simulink model "VEC"  (R2016a)
settings: Solver=ode45  SolverMode=SingleTasking  StartTime=0.0  StopTime=2000  FixedStep=0.001  RelTol=1e-5  AbsTol=1e-6
PostLoadFcn:
  | sldemo_fuelsys_data(bdroot,'initialize_data','orig','float');
model workspace (MAT data in the model file):
  PressEst = [0.806253176324 0.553142316929 0.37151500209 0.277667903103 0.220198954207 0.181288665766 0.153200000489 0.115431020872 0.0913067476324 0.0746519188607 0.0625231108324 0.0533383634277 ... (306 elements, 18x17)]
  PressVect = [0.05 0.1 0.15 0.2 0.25 0.3 0.35 0.4 0.45 0.5 0.55 0.6 0.65 0.7 0.75 0.8 0.85 0.9 0.95]
  PumpCon = [-0.0556348 -0.0022828 0.0256932 0.0435188 0.0562692 0.0661194857143 0.0741572 0.08697 0.0972452 0.106070342857 0.1139892 0.121303866667 ... (342 elements, 18x19)]
  RampRateKiX = [100 200 300 400 500 600]
  RampRateKiY = [0 0.2 0.4 0.6 0.8 1]
  RampRateKiZ = [0.012  0.024  0.036  0.048  0.06  0.072; 0.024  0.048  0.072  0.096  0.12  0.144; 0.036  0.072  0.108  0.144  0.18  0.216; 0.048  0.096  0.144  0.192  0.24  0.288; 0.06  0.12  0.18  0.24  0.3  0.36; 0.072  0.144  0.216  0.288  0.36  0.432]
  SpeedEst = [471.837839721 550.80940091 777.559313277 1080.9243499 1418.36795322 1769.7468768 2125.37309264 2480.20345067 2831.37796793 3177.14006959 3516.32917143 4064.90417867 ... (323 elements, 17x19)]
  SpeedVect = [50 75 100 125 150 175 200 250 300 350 400 450 500 600 700 800 900 1000]
  ThrotEst = [0 0 0 0 0 0 0 0 0 0 0 0 ... (342 elements, 18x19)]
  ThrotVect = [0 3 6 9 12 15 18 21 24 27 30 35 46 57 68 79 90]
  hys = 25
  max_ego = 1.2
  max_press = 0.95
  max_speed = 6000
  max_throt = 90
  min_press = 0.05
  min_speed = 50
  min_throt = 3
  st_range = 0.0001
  zero_thresh = 250
undefined symbols (not defined in the file): DiscIntNeverNeededParam, sld_FuelModes, sldvsubsys
libraries: simulink x4, simulink_extras x1
CloseFcn:
  | clear EngSensors u8En* s16En* sldemo_fuelsys_output
Description:
  | This is a model of a fuel control system where Stateflow(R) is used to handle the fault management of the system.
  | The system contains four separate sensors: a throttle sensor, a speed sensor, an oxygen sensor, and a pressure sensor.
  | Each of these sensors is represented by a parallel state in Stateflow.  Each parallel state contains two substates, a
  | normal state and a failed state (the exception being the oxygen sensor, which also contains a warmup state).
  | 
  | If any of the sensor readings is outside an acceptable range, then a fault is registered in Stateflow, and the
  | substate of the corresponding subsystem transitions to the failed state.  If a subsystem recovers, it can
  | transition back to the normal state.  The number of failures in the system at any given time is represented
  | in the Fail parallel state.
  | 
  | The last parallel state in the Stateflow chart is called Fueling_Mode.  This state regulates the oxygen to
  | fuel mixture ratio.  If a failure is detected, then the oxygen to fuel ratio is increased.  If multiple failures
  | are detected, then the fuel system is disabled until there are no longer multiple failures in the system.
settings Model: ModifiedByFormat=The MathWorks Inc.  NumberOfSteps=2  ExtModeTrigMode=oneshot  ExtModeArmWhenConnect=off  ExtModeAutoUpdateStatusClock=off  Creator=The MathWorks, Inc.  LastModifiedBy=The MathWorks Inc.
settings DataIOCC: SaveFormat=StructureWithTime  SaveOutput=off  SaveTime=off  SignalLoggingName=sldemo_fuelsys_output
settings OptimizationCC: DefaultParameterBehavior=Inlined  UseDivisionForNetSlopeComputation=UseDivisionForReciprocalsOfIntegersOnly  InlineInvariantSignals=on  EnhancedBackFolding=on  StrengthReduction=on  BooleansAsBitfields=on  PassReuseOutputArgsAs=Individual arguments  ExpressionDepthLimit=2147483647  ZeroExternalMemoryAtStartup=off  ZeroInternalMemoryAtStartup=off  NoFixptDivByZeroProtection=on  EfficientFloat2IntCast=on  OptimizeModelRefInitCode=on  LifeSpan=1
settings DebuggingCC: SignalInfNanChecking=error  SaveWithParameterizedLinksMsg=none  UnderspecifiedInitializationDetection=Classic  CheckExecutionContextPreStartOutputMsg=on  CheckExecutionContextRuntimeOutputMsg=on  IntegerOverflowMsg=none  ParameterDowncastMsg=warning  ParameterOverflowMsg=none  ParameterPrecisionLossMsg=none  UnderSpecifiedDataTypeMsg=warning  FcnCallInpInsideContextMsg=UseLocalSettings  UniqueDataStoreMsg=error  BusObjectLabelMismatch=error  AllowSymbolicDim=off  StateNameClashWarn=warning  StrictBusMsg=ErrorOnBusTreatedAsVector  IntegerSaturationMsg=none
settings HardwareCC: ProdBitPerPointer=32  ProdLargestAtomicFloat=None  ProdWordSize=32  ProdHWDeviceType=Specified
settings ModelReferenceCC: PropagateSignalLabelsOutOfModel=off
settings SFSimCC: SimParseCustomCode=off
settings RTWCC: SystemTargetFile=ert.tlc  TemplateMakefile=ert_default_tmf  Description=Real-Time Workshop Embedded Coder  GenerateReport=on  RTWVerbose=off  IncludeHyperlinkInReport=on  LaunchReport=on  GenerateTraceInfo=on  GenerateTraceReport=on  GenerateTraceReportSl=on  GenerateTraceReportSf=on  GenerateTraceReportEml=on
settings CodeAppCC: ForceParamTrailComments=on  IgnoreCustomStorageClasses=off  IgnoreTestpoints=on  SimulinkDataObjDesc=on  SFDataObjDesc=on  CustomSymbolStrGlobalVar=rt$N$M  CustomSymbolStrType=$N$M  CustomSymbolStrFcn=$N$M$F  CustomSymbolStrMacro=$N$M  InsertBlockDesc=on  InternalIdentifier=Classic  ReqsInCode=on
settings ERTTargetCC: GenerateSampleERTMain=on  IncludeMdlTerminateFcn=off  SupportAbsoluteTime=off  SupportNonFinite=off  SupportComplex=off  InlinedParameterPlacement=NonHierarchical  ERTCustomFileTemplate=example_file_process.tlc  ConvertIfToSwitch=off  SuppressUnreachableDefaultCases=off
settings ConfigComp: CovPath=/fuel_rate_control/control_logic  CovSFcnEnable=off

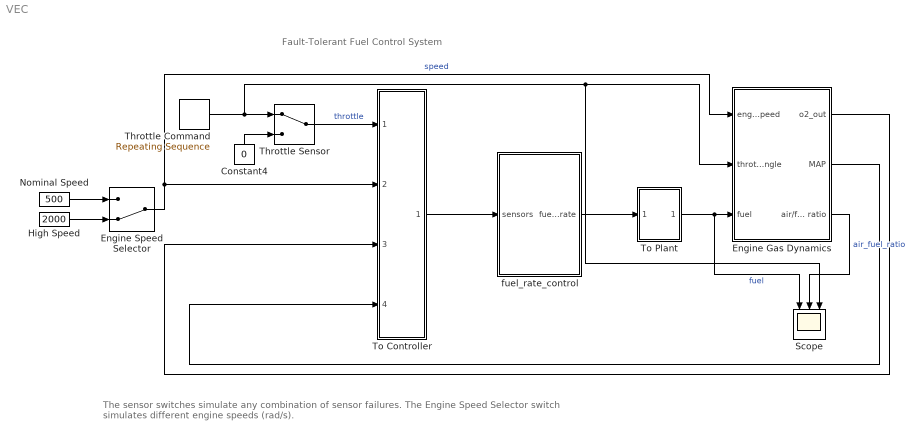
== system VEC ==
  note: Fault-Tolerant Fuel Control System
  note: The sensor switches simulate any combination of sensor failures.
      | The Engine Speed Selector switch simulates different engine speeds (rad/s).
  Constant4 : Constant  Value=0
  Engine Speed Selector : ManualSwitch  CurrentSetting=0
  Engine Gas Dynamics : Subsystem
  High Speed : Constant  Value=2000
  Nominal Speed : Constant  Value=500
  Scope : Scope  NumInputPorts=3
  Throttle Command : simulink/Sources/Repeating Sequence  rep_seq_t=[0 0.2 0.9 1]  rep_seq_y=[5 90 90 5]
  Throttle Sensor : ManualSwitch
  To Controller : Subsystem
      mask Display: fprintf('Convert')
  To Plant : Subsystem
      mask Display: fprintf('Convert')
  fuel_rate_control : Subsystem  Tag=FuelRateControl  TreatAsAtomicUnit=on
  wires:
  Engine Gas Dynamics/3(air/fuel ratio) -> Scope/2  "air_fuel_ratio"
  fuel_rate_control/1(fuel_rate) -> To Plant/1(In1)
  Engine Gas Dynamics/1(o2_out) -> To Controller/3(ego)
  Throttle Command/1 -> Scope/3, Engine Gas Dynamics/2(throttle angle), Throttle Sensor/1
  Constant4/1 -> Throttle Sensor/2
  Engine Gas Dynamics/2(MAP) -> To Controller/4(map)
  High Speed/1 -> Engine Speed Selector/2
  Nominal Speed/1 -> Engine Speed Selector/1
  Throttle Sensor/1 -> To Controller/1(throttle)  "throttle"
  Engine Speed Selector/1 -> To Controller/2(speed), Engine Gas Dynamics/1(engine speed)  "speed"
  To Plant/1(Out1) -> Scope/1, Engine Gas Dynamics/3(fuel)  "fuel"
  To Controller/1(sensors) -> fuel_rate_control/1(sensors)

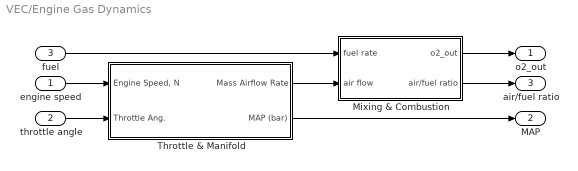
== system VEC/Engine Gas Dynamics ==
  engine speed : Inport  Unit=rad/s
  throttle angle : Inport  Port=2  Unit=deg
  fuel : Inport  Port=3  Unit=g/s
  Mixing & Combustion : Subsystem
  Throttle & Manifold : Subsystem
  o2_out : Outport  Unit=V
  MAP : Outport  Port=2  Unit=bar
  air/fuel ratio : Outport  Port=3  Unit=1
  wires:
  Throttle & Manifold/1(Mass Airflow Rate) -> Mixing & Combustion/2(air flow)
  fuel/1 -> Mixing & Combustion/1(fuel rate)
  engine speed/1 -> Throttle & Manifold/1("Engine Speed, N")
  throttle angle/1 -> Throttle & Manifold/2(Throttle Ang.)
  Mixing & Combustion/2(air/fuel ratio) -> air/fuel ratio/1
  Throttle & Manifold/2(MAP (bar)) -> MAP/1
  Mixing & Combustion/1(o2_out) -> o2_out/1

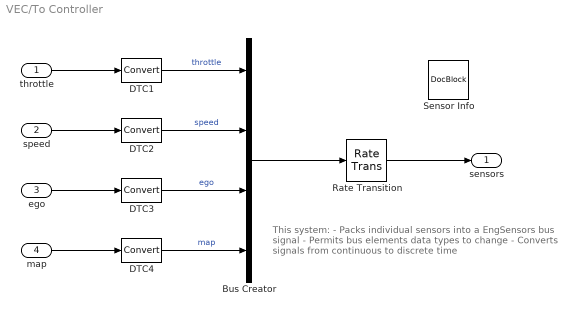
== system VEC/To Controller ==
  note: This system:
      | - Packs individual sensors into a EngSensors bus signal
      | - Permits bus elements data types to change
      | - Converts signals from continuous to discrete time
  throttle : Inport
  speed : Inport  Port=2
  ego : Inport  Port=3
  map : Inport  Port=4
  Bus Creator : BusCreator  Inputs=4  OutDataTypeStr=Bus: EngSensors  NonVirtualBus=on
  DTC{1..4} (4 alike) : DataTypeConversion  SampleTime=[0 1]
  Rate Transition : RateTransition  OutPortSampleTime=0.01
  Sensor Info : simulink/Model-Wide Utilities/DocBlock  DocumentType=Text
      content=|
      | Measurement Descriptions
      | ========================
      |
      | Throttle Angle (degrees):
      | min=3, max=90, precision=0.1
      |
      | Engine Speed (radians/sec.):
      | min=0, max=620, precision=.1
      |
      | Ego Sensor (volts):
      | min=0, max=12, precision=.05
      |
      | Manifold Pressure (bar):
      | min=0.001, max=1, precision=.001
  sensors : Outport
  wires:
  throttle/1 -> DTC1/1
  DTC1/1 -> Bus Creator/1  "throttle"
  speed/1 -> DTC2/1
  DTC2/1 -> Bus Creator/2  "speed"
  ego/1 -> DTC3/1
  DTC3/1 -> Bus Creator/3  "ego"
  map/1 -> DTC4/1
  DTC4/1 -> Bus Creator/4  "map"
  Bus Creator/1 -> Rate Transition/1
  Rate Transition/1 -> sensors/1

== system VEC/To Plant ==
  note: This system:
      | - Permits upstream signal data type to change
      | - Converts signals from discrete to continuous time
  In1 : Inport
  DTC5 : DataTypeConversion
  Rate Transition1 : RateTransition  Integrity=off  X0=1.6  OutPortSampleTime=0
  Out1 : Outport
  wires:
  DTC5/1 -> Rate Transition1/1
  In1/1 -> DTC5/1
  Rate Transition1/1 -> Out1/1

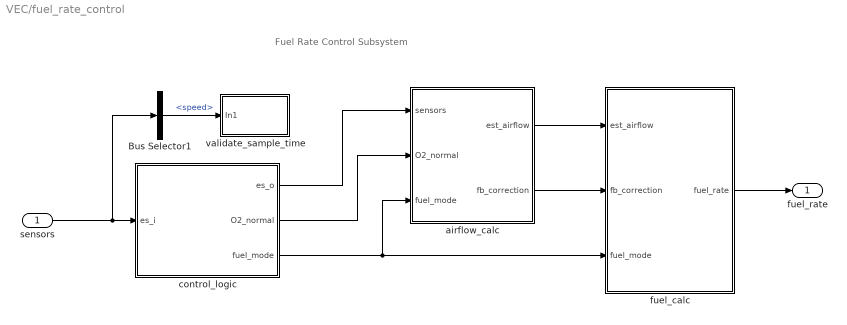
== system VEC/fuel_rate_control ==
  note: Fuel Rate Control Subsystem
  sensors : Inport  OutDataTypeStr=Bus: EngSensors
  Bus Selector1 : BusSelector  OutputSignals=speed
  airflow_calc : Subsystem
  control_logic : Stateflow chart  Description=Stateflow diagram to determine control system operating mode  TreatAsAtomicUnit=on
  fuel_calc : Subsystem
  validate_sample_time : Subsystem  Tag=VerificationSubsystem  DisableCoverage=on  LoadFcn=sldvsubsys('check')  TreatAsAtomicUnit=on  SimViewingDevice=on  mask(VerificationSubsystem){}
      mask init:
      | sldvsubsys('maskInit');
      settings: CopyFcn=sldvsubsys('copy');  OpenFcn=open_system(gcb,'force');
      settings: PreSaveFcn=|
      | set_param(gcb,'SimViewingDevice','on');
      | sldvsubsys('check');
      mask Help: helpview(fullfile(docroot,'toolbox','sldv','sldv.map'),'verificationsubsystem')
      mask Display: image(imread('sldvicon_versubsys.png','BackGroundColor',[1 1 1]),'center');
  fuel_rate : Outport  Unit=g/s
  wires:
  fuel_calc/1(fuel_rate) -> fuel_rate/1
  airflow_calc/1(est_airflow) -> fuel_calc/1(est_airflow)
  sensors/1 -> control_logic/1(es_i), Bus Selector1/1
  control_logic/3(fuel_mode) -> airflow_calc/3(fuel_mode), fuel_calc/3(fuel_mode)
  control_logic/1(es_o) -> airflow_calc/1(sensors)
  control_logic/2(" O2_normal") -> airflow_calc/2(O2_normal)
  airflow_calc/2(fb_correction) -> fuel_calc/2(fb_correction)
  Bus Selector1/1 -> validate_sample_time/1(In1)  "<speed>"

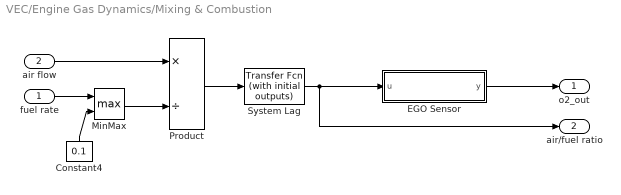
== system VEC/Engine Gas Dynamics/Mixing & Combustion ==
  fuel rate : Inport  Unit=g/s
  air flow : Inport  Port=2  Unit=g/s
  Constant4 : Constant  Value=0.1
  EGO Sensor : MATLAB Function  TreatAsAtomicUnit=on
  MinMax : MinMax  Function=max  Inputs=2  SaturateOnIntegerOverflow=on  InputSameDT=on
  Product : Product  Inputs=*/  SaturateOnIntegerOverflow=on  RndMeth=Zero  InputSameDT=on  OutDataTypeStr=Inherit: Same as first input
  System Lag : simulink_extras/Additional Linear/Transfer Fcn (with initial outputs)  N=3  D=[1 3]  Y0=1/14.6  U0=1/14.6
  o2_out : Outport  Unit=V
  air/fuel ratio : Outport  Port=2  Unit=1
  wires:
  Constant4/1 -> MinMax/2
  fuel rate/1 -> MinMax/1
  MinMax/1 -> Product/2
  Product/1 -> System Lag/1
  System Lag/1 -> air/fuel ratio/1, EGO Sensor/1(u)
  EGO Sensor/1(y) -> o2_out/1
  air flow/1 -> Product/1

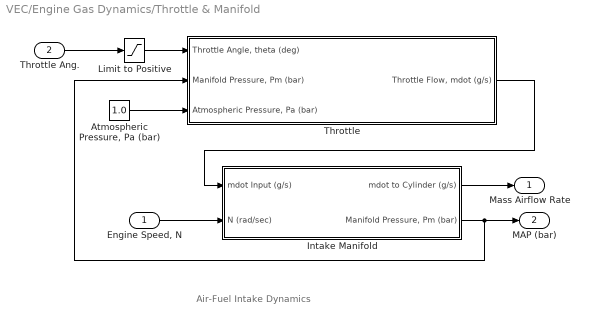
== system VEC/Engine Gas Dynamics/Throttle & Manifold ==
  note: Air-Fuel Intake Dynamics
  "Engine Speed, N" : Inport  Unit=rad/s
  Throttle Ang. : Inport  Port=2  Unit=deg
  "Atmospheric Pressure, Pa (bar)" : Constant  Value=1.0
  Intake Manifold : Subsystem
  Limit to Positive : Saturate  UpperLimit=inf  LowerLimit=0
  Throttle : Subsystem
  Mass Airflow Rate : Outport  Unit=g/s
  MAP (bar) : Outport  Port=2  Unit=bar
  wires:
  Limit to Positive/1 -> Throttle/1("Throttle Angle, theta (deg)")
  Throttle Ang./1 -> Limit to Positive/1
  Throttle/1("Throttle Flow, mdot (g/s)") -> Intake Manifold/1(mdot Input (g/s))
  "Engine Speed, N"/1 -> Intake Manifold/2(N (rad/sec))
  Intake Manifold/1(mdot to Cylinder (g/s)) -> Mass Airflow Rate/1
  "Atmospheric Pressure, Pa (bar)"/1 -> Throttle/3("Atmospheric Pressure, Pa (bar) ")
  Intake Manifold/2("Manifold Pressure, Pm (bar)") -> Throttle/2("Manifold Pressure, Pm (bar)"), MAP (bar)/1

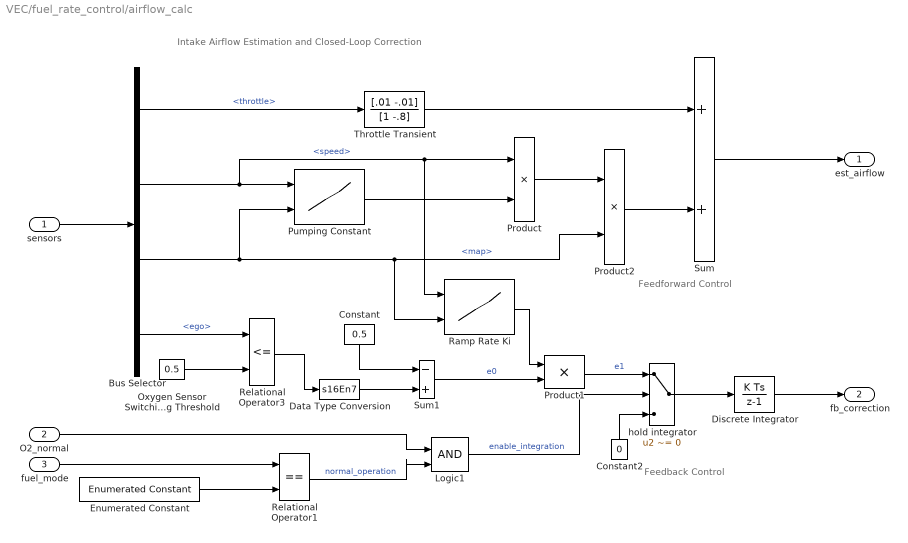
== system VEC/fuel_rate_control/airflow_calc ==
  note: Intake Airflow Estimation and Closed-Loop Correction
  note: Feedback Control
  note: Feedforward Control
  sensors : Inport
  O2_normal : Inport  Port=2
  fuel_mode : Inport  Port=3
  Bus Selector : BusSelector  OutputSignals=throttle,speed,map,ego
  Constant : Constant  Value=0.5  OutDataTypeStr=s16En7
  Constant2 : Constant  Value=0  OutDataTypeStr=uint8
  Data Type Conversion : DataTypeConversion  OutDataTypeStr=s16En7  RndMeth=Simplest
  Discrete Integrator : DiscreteIntegrator  InitialConditionSetting=State (most efficient)  SampleTime=-1  OutDataTypeStr=s16En15  RndMeth=Simplest  ICPrevOutput=DiscIntNeverNeededParam  ICPrevScaledInput=DiscIntNeverNeededParam
  Enumerated Constant : simulink/Sources/Enumerated Constant  OutDataTypeStr=Enum: sld_FuelModes  Value=sld_FuelModes.LOW  SampleTime=.01
  Logic1 : Logic  IconShape=distinctive  AllPortsSameDT=off  OutDataTypeStr=boolean
  Oxygen Sensor Switching Threshold : Constant  Value=0.5  OutDataTypeStr=s16En7
  Product : Product  OutDataTypeStr=s16En7  RndMeth=Simplest
  Product1 : Product  OutDataTypeStr=s16En15  RndMeth=Simplest
  Product2 : Product  OutDataTypeStr=s16En7  RndMeth=Simplest
  Pumping Constant : Lookup_n-D  BreakpointsForDimension1=SpeedVect  BreakpointsForDimension2=PressVect  IndexSearchMethod=Linear search  Table=PumpCon  ExtrapMethod=Clip  UseLastTableValue=on  OutDataTypeStr=s16En15  RndMeth=Simplest
  Ramp Rate Ki : Lookup_n-D  BreakpointsForDimension1=RampRateKiX  BreakpointsForDimension2=RampRateKiY  IndexSearchMethod=Linear search  Table=RampRateKiZ  ExtrapMethod=Clip  UseLastTableValue=on  OutDataTypeStr=s16En15  RndMeth=Simplest
  Relational Operator1 : RelationalOperator  Operator===  OutDataTypeStr=boolean  InputSameDT=on
  Relational Operator3 : RelationalOperator  Operator=<=  OutDataTypeStr=boolean
  Sum : Sum  Inputs=2  OutDataTypeStr=s16En7  RndMeth=Simplest
  Sum1 : Sum  Inputs=-+  OutDataTypeStr=s16En15  RndMeth=Simplest
  Throttle Transient : DiscreteFilter  Numerator=[.01 -.01]  Denominator=[1 -.8]  a0EqualsOne=on  OutDataTypeStr=s16En7  RndMeth=Simplest
  hold integrator : Switch  Criteria=u2 ~= 0  Threshold=1  OutDataTypeStr=s16En15  RndMeth=Simplest
  est_airflow : Outport  Unit=g/s
  fb_correction : Outport  Port=2
  wires:
  Discrete Integrator/1 -> fb_correction/1
  sensors/1 -> Bus Selector/1
  Pumping Constant/1 -> Product/2
  Bus Selector/2 -> Product/1, Ramp Rate Ki/1, Pumping Constant/1  "<speed>"
  Throttle Transient/1 -> Sum/1
  Sum/1 -> est_airflow/1
  Bus Selector/1 -> Throttle Transient/1  "<throttle>"
  Relational Operator1/1 -> Logic1/2  "normal_operation"
  Oxygen Sensor Switching Threshold/1 -> Relational Operator3/2
  Constant/1 -> Sum1/1
  Ramp Rate Ki/1 -> Product1/1
  Constant2/1 -> hold integrator/3
  Product1/1 -> hold integrator/1  "e1"
  hold integrator/1 -> Discrete Integrator/1
  Logic1/1 -> hold integrator/2  "enable_integration"
  Sum1/1 -> Product1/2  "e0"
  Relational Operator3/1 -> Data Type Conversion/1
  Data Type Conversion/1 -> Sum1/2
  Bus Selector/3 -> Product2/2, Ramp Rate Ki/2, Pumping Constant/2  "<map>"
  Bus Selector/4 -> Relational Operator3/1  "<ego>"
  Product/1 -> Product2/1
  Product2/1 -> Sum/2
  O2_normal/1 -> Logic1/1
  Enumerated Constant/1 -> Relational Operator1/2
  fuel_mode/1 -> Relational Operator1/1

== system VEC/fuel_rate_control/control_logic/Pressure.map_estimate ==
  note: MAP Estimation
  speed : Inport  OutDataTypeStr=s16En3
  throttle : Inport  Port=2  OutDataTypeStr=s16En3
  f : TriggerPort  TriggerType=function-call  VariantControl=Variant
      settings: CopyFcn=Stateflow.SLINSF.SimulinkMan.removeBlockPreDeleteFcn  PreDeleteFcn=Stateflow.SLINSF.SimulinkMan.unsafePredeleteFcn
  Pressure Estimation : Lookup_n-D  BreakpointsForDimension1=SpeedVect  BreakpointsForDimension2=ThrotVect  IndexSearchMethod=Linear search  Table=PressEst  ExtrapMethod=Clip  UseLastTableValue=on  OutDataTypeStr=u8En7  RndMeth=Simplest
  map : Outport
  wires:
  speed/1 -> Pressure Estimation/1
  throttle/1 -> Pressure Estimation/2
  Pressure Estimation/1 -> map/1

== system VEC/fuel_rate_control/control_logic/Speed.speed_estimate ==
  note: Speed Estimation
  throttle : Inport  OutDataTypeStr=s16En3
  map : Inport  Port=2  OutDataTypeStr=u8En7
  f : TriggerPort  TriggerType=function-call  VariantControl=Variant
      settings: CopyFcn=Stateflow.SLINSF.SimulinkMan.removeBlockPreDeleteFcn  PreDeleteFcn=Stateflow.SLINSF.SimulinkMan.unsafePredeleteFcn
  Saturation : Saturate  UpperLimit=max_speed  LowerLimit=0  OutDataTypeStr=s16En3
  Speed Estimation : Lookup_n-D  BreakpointsForDimension1=ThrotVect  BreakpointsForDimension2=PressVect  IndexSearchMethod=Linear search  Table=SpeedEst  ExtrapMethod=Clip  UseLastTableValue=on  OutDataTypeStr=s16En3  RndMeth=Simplest
  speed : Outport
  wires:
  Speed Estimation/1 -> Saturation/1
  throttle/1 -> Speed Estimation/1
  map/1 -> Speed Estimation/2
  Saturation/1 -> speed/1

== system VEC/fuel_rate_control/control_logic/Throttle.throttle_estimate ==
  note: Throttle Estimation
  speed : Inport  OutDataTypeStr=s16En3
  map : Inport  Port=2  OutDataTypeStr=u8En7
  f : TriggerPort  TriggerType=function-call  VariantControl=Variant
      settings: CopyFcn=Stateflow.SLINSF.SimulinkMan.removeBlockPreDeleteFcn  PreDeleteFcn=Stateflow.SLINSF.SimulinkMan.unsafePredeleteFcn
  Throttle Estimation : Lookup_n-D  BreakpointsForDimension1=SpeedVect  BreakpointsForDimension2=PressVect  IndexSearchMethod=Linear search  Table=ThrotEst  ExtrapMethod=Clip  UseLastTableValue=on  OutDataTypeStr=s16En7  RndMeth=Simplest
  throttle : Outport
  wires:
  speed/1 -> Throttle Estimation/1
  map/1 -> Throttle Estimation/2
  Throttle Estimation/1 -> throttle/1

== system VEC/fuel_rate_control/fuel_calc ==
  note: Fuel Rate Calculation
  est_airflow : Inport  Unit=g/s
  fb_correction : Inport  Port=2
  fuel_mode : Inport  Port=3
  feedforward_fuel_rate : Subsystem
  switchable_compensation : Subsystem
  fuel_rate : Outport  Unit=g/s
  wires:
  est_airflow/1 -> feedforward_fuel_rate/1(est_airflow)
  fuel_mode/1 -> feedforward_fuel_rate/2(fuel_mode), switchable_compensation/2(fuel_mode)
  switchable_compensation/1(fuel_rate) -> fuel_rate/1
  fb_correction/1 -> switchable_compensation/3(fb_correction)
  feedforward_fuel_rate/1(ff_fuel_rate) -> switchable_compensation/1(ff_fuel_rate)

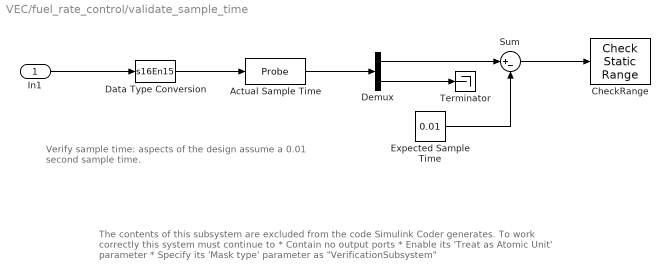
== system VEC/fuel_rate_control/validate_sample_time ==
  note: The contents of this subsystem are excluded from the code Simulink Coder generates.
      |
      | To work correctly this system must continue to
      | * Contain no output ports
      | * Enable its 'Treat as Atomic Unit' parameter
      | * Specify its 'Mask type' parameter as "VerificationSubsystem"
  note: Verify sample time: aspects of the design
      | assume a 0.01 second sample time.
  In1 : Inport
  Actual Sample Time : Probe  ProbeWidth=off  ProbeComplexSignal=off  ProbeSampleTimeDataType=Same as input
  CheckRange : simulink/Model Verification/Check  Static Range  Description=-st_range < u < st_range  max=st_range  max_included=off  min=-st_range  min_included=off  enabled=on  stopWhenAssertionFail=on  export=off  icon=graphic
  Data Type Conversion : DataTypeConversion  OutDataTypeStr=s16En15
  Demux : Demux  Outputs=2
  Expected Sample Time : Constant  Value=0.01  OutDataTypeStr=s16En15
  Sum : Sum  Inputs=|+-  OutDataTypeStr=Inherit: Same as first input
  Terminator : Terminator
  wires:
  Actual Sample Time/1 -> Demux/1
  In1/1 -> Data Type Conversion/1
  Demux/2 -> Terminator/1
  Demux/1 -> Sum/1
  Expected Sample Time/1 -> Sum/2
  Sum/1 -> CheckRange/1
  Data Type Conversion/1 -> Actual Sample Time/1

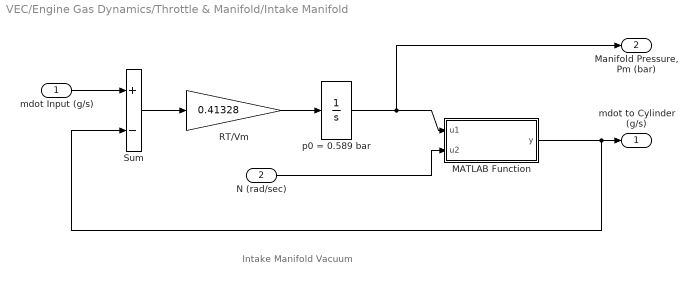
== system VEC/Engine Gas Dynamics/Throttle & Manifold/Intake Manifold ==
  note: Intake Manifold Vacuum
  mdot Input (g/s) : Inport  Unit=g/s
  N (rad/sec) : Inport  Port=2  Unit=rad/s
  MATLAB Function : MATLAB Function  TreatAsAtomicUnit=on
  RT/Vm : Gain  Gain=0.41328  SaturateOnIntegerOverflow=on  OutDataTypeStr=Inherit: Same as input  ParamDataTypeStr=Inherit: Same as input
  Sum : Sum  Inputs=+-  SaturateOnIntegerOverflow=on  InputSameDT=on  OutDataTypeStr=Inherit: Same as first input
  p0 = 0.589 bar : Integrator  InitialCondition=.589
  mdot to Cylinder (g/s) : Outport  Unit=g/s
  "Manifold Pressure, Pm (bar)" : Outport  Port=2  Unit=bar
  wires:
  mdot Input (g/s)/1 -> Sum/1
  RT/Vm/1 -> p0 = 0.589 bar/1
  N (rad/sec)/1 -> MATLAB Function/2(u2)
  p0 = 0.589 bar/1 -> "Manifold Pressure, Pm (bar)"/1, MATLAB Function/1(u1)
  Sum/1 -> RT/Vm/1
  MATLAB Function/1(y) -> mdot to Cylinder (g/s)/1, Sum/2

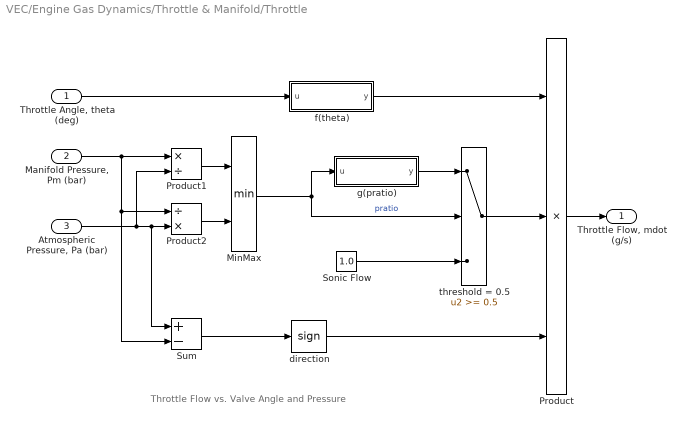
== system VEC/Engine Gas Dynamics/Throttle & Manifold/Throttle ==
  note: Throttle Flow vs. Valve Angle and Pressure
  "Throttle Angle, theta (deg)" : Inport  Unit=deg
  "Manifold Pressure, Pm (bar)" : Inport  Port=2  Unit=bar
  "Atmospheric Pressure, Pa (bar) " : Inport  Port=3  Unit=bar
  MinMax : MinMax  Inputs=2  SaturateOnIntegerOverflow=on  InputSameDT=on
  Product : Product  Inputs=3  SaturateOnIntegerOverflow=on  RndMeth=Zero  InputSameDT=on  OutDataTypeStr=Inherit: Same as first input
  Product1 : Product  Inputs=*/  SaturateOnIntegerOverflow=on  RndMeth=Zero  InputSameDT=on  OutDataTypeStr=Inherit: Same as first input
  Product2 : Product  Inputs=/*  SaturateOnIntegerOverflow=on  RndMeth=Zero  InputSameDT=on  OutDataTypeStr=Inherit: Same as first input
  "Sonic Flow " : Constant  Value=1.0
  Sum : Sum  Inputs=+-  SaturateOnIntegerOverflow=on  InputSameDT=on  OutDataTypeStr=Inherit: Same as first input
  direction : Signum
  f(theta) : MATLAB Function  TreatAsAtomicUnit=on
  g(pratio) : MATLAB Function  TreatAsAtomicUnit=on
  threshold = 0.5 : Switch  Threshold=0.5  SaturateOnIntegerOverflow=on  InputSameDT=on
  "Throttle Flow, mdot (g/s)" : Outport  Unit=g/s
  wires:
  "Manifold Pressure, Pm (bar)"/1 -> Sum/2, Product2/1, Product1/1
  Product2/1 -> MinMax/2
  Product1/1 -> MinMax/1
  "Atmospheric Pressure, Pa (bar) "/1 -> Sum/1, Product2/2, Product1/2
  g(pratio)/1(y) -> threshold = 0.5/1
  "Sonic Flow "/1 -> threshold = 0.5/3
  threshold = 0.5/1 -> Product/2
  direction/1 -> Product/3
  Sum/1 -> direction/1
  MinMax/1 -> threshold = 0.5/2, g(pratio)/1(u)  "pratio"
  "Throttle Angle, theta (deg)"/1 -> f(theta)/1(u)
  Product/1 -> "Throttle Flow, mdot (g/s)"/1
  f(theta)/1(y) -> Product/1

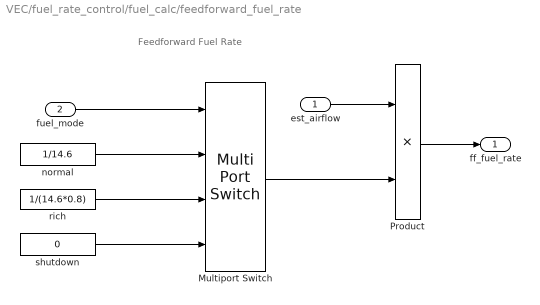
== system VEC/fuel_rate_control/fuel_calc/feedforward_fuel_rate ==
  note: Feedforward Fuel Rate
  est_airflow : Inport
  fuel_mode : Inport  Port=2
  Multiport Switch : MultiPortSwitch  DataPortOrder=Specify indices  DataPortIndices={sld_FuelModes.LOW, sld_FuelModes.RICH, sld_FuelModes.DISABLED}  OutDataTypeStr=s16En7  RndMeth=Simplest
  Product : Product  OutDataTypeStr=s16En7  RndMeth=Simplest
  normal : Constant  Value=1/14.6  OutDataTypeStr=s16En7
  rich : Constant  Value=1/(14.6*0.8)  OutDataTypeStr=s16En7
  shutdown : Constant  Value=0  OutDataTypeStr=s16En7
  ff_fuel_rate : Outport
  wires:
  rich/1 -> Multiport Switch/3
  fuel_mode/1 -> Multiport Switch/1
  est_airflow/1 -> Product/1
  Product/1 -> ff_fuel_rate/1
  Multiport Switch/1 -> Product/2
  normal/1 -> Multiport Switch/2
  shutdown/1 -> Multiport Switch/4

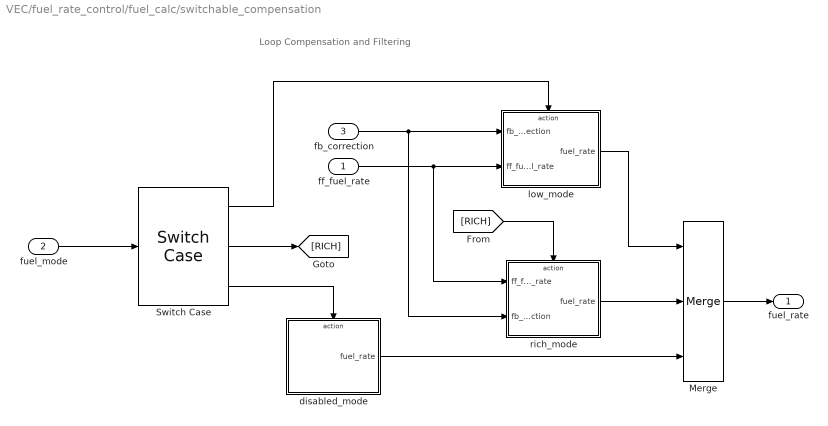
== system VEC/fuel_rate_control/fuel_calc/switchable_compensation ==
  note: Loop Compensation and Filtering
  ff_fuel_rate : Inport
  fuel_mode : Inport  Port=2
  fb_correction : Inport  Port=3
  Merge : Merge  Inputs=3
  Switch Case : SwitchCase  CaseConditions={sld_FuelModes.LOW, sld_FuelModes.RICH}
  disabled_mode : Subsystem  TreatAsAtomicUnit=on
  low_mode : Subsystem  TreatAsAtomicUnit=on
  rich_mode : Subsystem  TreatAsAtomicUnit=on
  fuel_rate : Outport
  wires:
  fuel_mode/1 -> Switch Case/1
  ff_fuel_rate/1 -> rich_mode/1(ff_fuel_rate), low_mode/2(ff_fuel_rate)
  fb_correction/1 -> rich_mode/2(fb_correction), low_mode/1(fb_correction)
  Switch Case/1 -> low_mode/Action
  Switch Case/2 -> [RICH]
  [RICH] -> rich_mode/Action
  Switch Case/3 -> disabled_mode/Action
  rich_mode/1(fuel_rate) -> Merge/2
  disabled_mode/1(fuel_rate) -> Merge/3
  low_mode/1(fuel_rate) -> Merge/1
  Merge/1 -> fuel_rate/1

== system VEC/fuel_rate_control/fuel_calc/switchable_compensation/disabled_mode ==
  note: Disabled Mode Fuel Mode
  Action Port : ActionPort  ActionType=default
  shutoff : Constant  Value=0  OutDataTypeStr=Inherit: Inherit via back propagation
  fuel_rate : Outport  InitialOutput=0
  wires:
  shutoff/1 -> fuel_rate/1

== system VEC/fuel_rate_control/fuel_calc/switchable_compensation/low_mode ==
  note: Low Mode Fuel Mode
  fb_correction : Inport
  ff_fuel_rate : Inport  Port=2
  Action Port : ActionPort  ActionType=case
  Discrete Filter : DiscreteFilter  Numerator=[8.7696 -8.5104]  Denominator=[1 -0.7408]  a0EqualsOne=on  RndMeth=Simplest  OutDataTypeStr=Inherit: Same as input
  Sum3 : Sum  OutDataTypeStr=s16En7  RndMeth=Simplest
  fuel_rate : Outport  InitialOutput=0
  wires:
  ff_fuel_rate/1 -> Sum3/2
  Discrete Filter/1 -> Sum3/1
  Sum3/1 -> fuel_rate/1
  fb_correction/1 -> Discrete Filter/1

== system VEC/fuel_rate_control/fuel_calc/switchable_compensation/rich_mode ==
  note: Rich Mode Fuel Mode
  ff_fuel_rate : Inport
  fb_correction : Inport  Port=2
  Action Port : ActionPort  ActionType=case
  Discrete Filter : DiscreteFilter  Numerator=[0 0.2592]  Denominator=[1 -0.7408]  a0EqualsOne=on  RndMeth=Simplest  OutDataTypeStr=Inherit: Same as input
  Sum2 : Sum  OutDataTypeStr=s16En7  RndMeth=Simplest
  fuel_rate : Outport  InitialOutput=0
  wires:
  fb_correction/1 -> Sum2/2
  ff_fuel_rate/1 -> Sum2/1
  Sum2/1 -> Discrete Filter/1
  Discrete Filter/1 -> fuel_rate/1

== stateflow chart VEC/fuel_rate_control/control_logic ==
  state O2 [parallel]
    settings: executionOrder=1  description=This state determines the validity of the exhaust gas oxygen sensor (EGO) data.
    state A
      du:
      es_o.ego = es_i.ego;
      state O2_warmup
        settings: description=The EGO sensor must come up to temperature before its data is reliable.
      state O2_normal
        settings: description=Normal EGO sensor operation gives a reliable indication of excess oxygen in the exhaust gas, from which air/fuel mixture can be inferred.
      state O2_failure
        settings: description=The EGO sensor has failed.
      (default) -> O2_warmup
      O2_warmup -> O2_normal : [after(480,tick)]
        settings: description=The value for sufficient warm up to operational temperature (nominally 4.8 seconds).
      O2_failure -> O2_normal : [es_i.ego < max_ego] / Fail.DEC;
      O2_normal -> O2_failure : [es_i.ego > max_ego] / Fail.INC;
        settings: description=The failure condition is indicated by excessive output voltage.
    (default) -> A
  state Pressure [parallel]
    settings: executionOrder=2  description=This state assesses the validity of the manifold absolute pressure (MAP) sensor.
    state normal
      du:
      es_o.map = es_i.map;
      settings: description=The manifold pressure sensor gives a reliable indication of absolute pressure (MAP).
    state fail
      du:
      es_o.map = map_estimate(es_i.speed, es_i.throttle);
      settings: description=The pressure sensor (manifold, or MAP) no longer produces reliable data.
    state map = map_estimate(speed, throttle) [function]
    (default) -> Pressure.normal
    Pressure.fail -> Pressure.normal : [es_i.map > min_press & ...
        | es_i.map < max_press] /
        | Fail.DEC;
    Pressure.normal -> Pressure.fail : [es_i.map > max_press | ...
        | es_i.map < min_press] /
        | Fail.INC;
  state Throttle [parallel]
    settings: executionOrder=3  description=This state determines the validity of the throttle sensor signal.
    state normal
      du:
      es_o.throttle = es_i.throttle;
      settings: description=The throttle sensor gives a reliable indication of the angle of the throttle plate.
    state fail
      du:
      es_o.throttle = throttle_estimate(es_i.speed,es_i.map);
      settings: description=Signal levels indicate that the throttle sensor data is no longer valid.
    state throttle = throttle_estimate(speed, map) [function]
    (default) -> Throttle.normal
    Throttle.fail -> Throttle.normal : [es_i.throttle >  min_throt & ...
        | es_i.throttle < max_throt] /
        | Fail.DEC;
    Throttle.normal -> Throttle.fail : [es_i.throttle> max_throt | ...
        | es_i.throttle < min_throt] /
        | Fail.INC;
      settings: description=A failure is indicated by data which is outside the expected range, typically due to an open or short circuit.
  state Speed [parallel]
    settings: executionOrder=4  description="This state infers the validity of the speed sensor data.  A failure is indicated by the presence of manifold vacuum at zero speed."
    state normal
      du:
      es_o.speed = es_i.speed;
      settings: description=The speed sensor data accurately represents the engine speed.
    state fail
      du:
      es_o.speed = speed_estimate(es_i.throttle, es_i.map);
      settings: description=The engine speed data is no longer available.
    state speed = speed_estimate(throttle, map) [function]
    (default) -> Speed.normal
    Speed.fail -> Speed.normal : [es_i.speed > 0C] /
        | Fail.DEC;
    Speed.normal -> Speed.fail : [es_i.speed == 0C & ...
        | es_i.map < zero_thresh] /
        | Fail.INC;
      settings: description="Loss of a reliable speed sensor signal will indicate zero speed.  This is deemed invalid when the manifold vacuum indicates otherwise."
  state Fail [parallel]
    settings: executionOrder=5  description=This state maintains a count of the number of sensors in failure mode.
    state Multi
      settings: description=This state represents any of the conditions in which more than one sensor is in failure mode.
      state Three
        settings: description=Three of the engine sensors have failed.
      state Four
        settings: description=All four of the engine sensors have failed.
      state Two
        settings: description=Two of the engine sensors have failed.
      Three -> Four [order 1] : INC
      Two -> Three [order 2] : INC
      Four -> Three : DEC
      Three -> Two [order 2] : DEC
    state One
      settings: description=One of the engine sensors has failed.
    state None
      settings: description=Zero failures; all sensors are operational.
    (default) -> None
    None -> One : INC
    One -> Two [order 1] : INC
    Two -> One [order 1] : DEC
    One -> None [order 2] : DEC
  state Fueling_Mode [parallel]
    settings: executionOrder=6  description=This state interprets the other states in the chart to directly control the fueling mode.
    state Fuel_Disabled
      en:
      fuel_mode = DISABLED;
      settings: description=The fuel is completely shut off while in this state.
      state Overspeed
        settings: description=The speed is dangerously high, so shut off the fuel.
      state Shutdown
        settings: description=Cut off system operation due to multiple sensor failures.
      Overspeed -> (junction 67) : [in(Speed.normal) & ...
          | es_i.speed < (max_speed - hys)]
      (junction 67) -> Shutdown [order 2] : [in(Fail.Multi)]
    state Running
      settings: description=The fuel is actively controlled while in this state.
      (history)
      state Low_Emissions
        en:
        fuel_mode = LOW;
        (history)
        state Warmup
          settings: description="The sensors are all operational, but the oxygen (EGO) sensor is warming up.  We'll target a stoichiometric ratio, nonetheless, but won't close the loop around exhaust gas oxygen."
        state Normal
          settings: description=All sensors are in correct operating modes, so effective closed-loop mixture control can be used.
        Warmup -> (junction 68) : [in(O2.A.O2_normal)]
        (junction 68) -> Normal [order 2]
      state Rich_Mixture
        en:
        fuel_mode = RICH;
        settings: description=This mode enriches the mixture, lowering the air/fuel ratio.
        state Single_Failure
          settings: description=Continue uninterrupted engine operation, but with a richer mixture.
      (junction 68) -> Single_Failure [order 1] : [in(Fail.One)]
      Normal -> Single_Failure : [in(Fail.One)]
      Single_Failure -> Normal : [in(Fail.None)]
    (default) -> Warmup : {es_o = es_i;}
      settings: description=Need to copy the sensors to the output on entry since the individual elements of the bus signal are only updated in the during function.
    Running -> Overspeed [order 2] : [es_i.speed > max_speed]
    (junction 67) -> Running [order 1] : [!in(Fail.Multi)]
    Running -> Shutdown [order 1] : enter(Fail.Multi)
    Shutdown -> Rich_Mixture : exit(Fail.Multi)
  data: speed function_input s16En3; throttle function_input s16En3; map function_output; speed function_input s16En3; map function_input u8En7; throttle function_output; throttle function_input s16En3; map function_input u8En7; speed function_output; es_o output EngSensors; O2_normal output boolean; max_ego parameter s16En7 [0..2]; max_press parameter u8En7 [0..2]; min_press parameter u8En7 [0..2]; min_throt parameter s16En3 [0..120]; max_throt parameter s16En3 [0..120]; zero_thresh parameter u8En7 [0..450]; max_speed parameter s16En3 [0..1000]; hys parameter s16En3 [0..1000]; es_i input EngSensors; fuel_mode output Enum: sld_FuelModes [1..3] =sld_FuelModes.LOW
  data es_o settings: description=Bus containing the sensor data.
  data max_ego settings: description=Parameter represents the upper end of the EGO sensor range.
  data max_press settings: description=Parameter represents the upper limt of valid pressure readings.
  data min_press settings: description=Parameter for the lower end of the valid pressure sensor range.
  data min_throt settings: description=Minimum valid throttle angle.
  data max_throt settings: description=Parameter to indicate the maximum valid throttle angle reading.
  data zero_thresh settings: description=Minimum manifold pressure expected at zero speed.
  data max_speed settings: description=Parameter for the upper end of the safe engine speed range.
  data hys settings: description=Hysteresis in the upper speed limit to avoid chatter at the threshold.
  data es_i settings: description=Bus containing the sensor data.
  data fuel_mode settings: description=Fuel control mode: LOW = stoichiometric mixture, RICH = rich mixture, DISABLED = shut down
  events: DEC local EITHER_EDGE_EVENT; INC local EITHER_EDGE_EVENT

== matlab function VEC/Engine Gas Dynamics/Throttle & Manifold/Throttle/f(theta) ==
  data: u input; y output
function y = f(u)
%#codegen

y = 2.821 - 0.05231*u + 0.10299*u^2 - 0.00063*u^3;

== matlab function VEC/Engine Gas Dynamics/Throttle & Manifold/Throttle/g(pratio) ==
  data: u input; y output
function y = g(u)
%#codegen

y = 2*sqrt(u - u^2);

== matlab function VEC/Engine Gas Dynamics/Throttle & Manifold/Intake Manifold/MATLAB Function ==
  data: u1 input; y output; u2 input
function y = pumping(u1,u2)
%#codegen

y = -0.366 + 0.08979*u1*u2 - 0.0337*u2*u1^2 + 0.0001*u1*u2^2;

== matlab function VEC/Engine Gas Dynamics/Mixing & Combustion/EGO Sensor ==
  data: u input; y output
function y = fcn(u)
%#codegen

y = (1-tanh(4*(u-14.6)))/2;
